simulink model "AMCLIB_FWSpeedLoop_BAM"  (Simulink 9.3)
settings: Solver=VariableStepAuto  StartTime=0.0  StopTime=10.0  RelTol=1e-3
(part 1 of 2)
settings Model: Creator=nxa18952  LastModifiedBy=nxa18952
settings DataIOCC: SaveFormat=Dataset  SignalLoggingSaveFormat=Dataset  ReturnWorkspaceOutputs=on
settings OptimizationCC: LifeSpan=auto
settings DebuggingCC: UnderspecifiedInitializationDetection=Simplified  MergeDetectMultiDrivingBlocksExec=error  FcnCallInpInsideContextMsg=error  SFUnexpectedBacktrackingDiag=error  SFNoUnconditionalDefaultTransitionDiag=error  SFExecutionAtInitializationDiag=warning  ArithmeticOperatorsInVariantConditions=error
settings HardwareCC: ProdBitPerPointer=64  ProdBitPerSizeT=64  ProdBitPerPtrDiffT=64  ProdLargestAtomicFloat=Float  ProdIntDivRoundTo=Zero  ProdEndianess=LittleEndian  ProdWordSize=64  ProdHWDeviceType=Intel->x86-64 (Windows64)
settings ModelReferenceCC: PropagateSignalLabelsOutOfModel=on
settings SFSimCC: SimUseLocalCustomCode=on
settings RTWCC: RTWUseLocalCustomCode=on
settings CodeAppCC: StateflowObjectComments=off
settings GRTTargetCC: TargetLangStandard=C99 (ISO)  CombineOutputUpdateFcns=on  GRTInterface=off
settings ConfigComp: CovMetricSettings=dwe  CovHtmlReporting=off  CovSaveCumulativeToWorkspaceVar=off  CovSaveSingleToWorkspaceVar=off  CovExternalEMLEnable=on

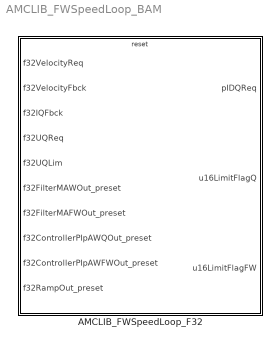
== system AMCLIB_FWSpeedLoop_BAM ==
  AMCLIB_FWSpeedLoop_F32 : Subsystem  TreatAsAtomicUnit=on  mask(AMCLIB_FWSpeedLoop_F32){showStates=Hide (faster execution), resetStatesEnable=Pre-set according to the first set of inputs after reset, showDebugOutputs=Hide, u16NSamplesW=0, u16NSamplesFW=0, f32PropGainQ=0, f32IntegGainQ=0, s16PropGainShiftQ=0, s16IntegGainShiftQ=0, f32LowerLimitQ=0, f32UpperLimitQ=0, f32PropGainFW=0, f32IntegGainFW=0, s16PropGainShiftFW=0, s16IntegGainShiftFW=0, f32LowerLimitFW=0, f32UpperLimitFW=0, f32RampUp=0, f32RampDown=0}
      mask prompts: showStates "Show internal states"; resetStatesEnable "Internal state after reset"; showDebugOutputs "Show debugging outputs"; u16NSamplesW "u16NSamplesW (velocity GDFLIB_FilterMA - recalculated smoothing factor)"; u16NSamplesFW "u16NSamplesFW (FW GDFLIB_FilterMA - recalculated smoothing factor)"; f32PropGainQ "f32PropGainQ (q-axis GFLIB_ControllerPIpAW - proportional gain)"; f32IntegGainQ "f32IntegGainQ (q-axis GFLIB_ControllerPIpAW - integral gain)"; s16PropGainShiftQ "s16PropGainShiftQ (q-axis GFLIB_ControllerPIpAW - scaling bitwise shift applied to the proportional gain)"; s16IntegGainShiftQ "s16IntegGainShiftQ (q-axis GFLIB_ControllerPIpAW - scaling bitwise shift applied to the integral gain)"; f32LowerLimitQ "f32LowerLimitQ (q-axis GFLIB_ControllerPIpAW - lower limit)"; f32UpperLimitQ "f32UpperLimitQ (q-axis GFLIB_ControllerPIpAW - upper limit)"; f32PropGainFW "f32PropGainFW (FW GFLIB_ControllerPIpAW - proportional gain)"; f32IntegGainFW "f32IntegGainFW (FW GFLIB_ControllerPIpAW - integral gain)"; s16PropGainShiftFW "s16PropGainShiftFW (FW GFLIB_ControllerPIpAW - scaling bitwise shift applied to the proportional gain)"; s16IntegGainShiftFW "s16IntegGainShiftFW (FW GFLIB_ControllerPIpAW - scaling bitwise shift applied to the integral gain)"; f32LowerLimitFW "f32LowerLimitFW (FW GFLIB_ControllerPIpAW - lower limit)"; f32UpperLimitFW "f32UpperLimitFW (FW GFLIB_ControllerPIpAW - upper limit)"; f32RampUp "f32RampUp (Ramp up increment coefficient)"; f32RampDown "f32RampDown (Ramp decrement coefficient)"
      mask help: Speed loop controller with Field Weakening capability for the PMSM field-oriented control algorithm in 32-bit fixed-point fractional implementation. This block supports re-initialization of the internal state during simulation. If the block is reset, the outputs of the MA filters, PI controllers, and the ramp will be aligned with the inputs f32FilterMAWOut_preset, f32FilterMAFWOut_preset, f32ControllerPIpAWQOut_preset, f32ControllerPIpAWFWOut_preset, and f32RampOut_preset. Refer to the AMMCLIB User's Guide for further details.
      mask init:
      | if ~evalin('base','exist(''tS8'',''var'')')
      |   if (2 ~= exist('SWLIBS_Typedefs.mat','file'))
      |       error('File SWLIBS_Typedefs.mat is not on the Matlab path. Please add the AMMCLIB "bam" folder in the Matlab Search Path.');
      |   else
      |       evalin('base', 'load(''SWLIBS_Typedefs.mat'')');
      |   end
      | end
      | if showStates == 1
      |     % hidden state variables
      |     if strcmp(get_param([gcb '/u16NSamplesW'], 'BlockType'), 'Inport')
      |         posblk = get_param(gcb, 'Position');
      | 
      |         pos = get_param(    [gcb, '/u16NSamplesW'], 'Position');
      |         orient = get_param( [gcb, '/u16NSamplesW'], 'Orientation');
      |         delete_block(       [gcb, '/u16NSamplesW']);
      |         add_block('built-in/Ground', [gcb, '/u16NSamplesW'], 'Position', pos, 'Orientation', orient);
      | 
      |         pos = get_param(    [gcb, '/u16NSamplesFW'], 'Position');
      |         orient = get_param( [gcb, '/u16NSamplesFW'], 'Orientation');
      |         delete_block(       [gcb, '/u16NSamplesFW']);
      |         add_block('built-in/Ground', [gcb, '/u16NSamplesFW'], 'Position', pos, 'Orientation', orient);
      | 
      |         pos = get_param(    [gcb, '/f32PropGainQ'], 'Position');
      |         orient = get_param( [gcb, '/f32PropGainQ'], 'Orientation');
      |         delete_block(       [gcb, '/f32PropGainQ']);
      |         add_block('built-in/Ground', [gcb, '/f32PropGainQ'], 'Position', pos, 'Orientation', orient);
      | 
      |         pos = get_param(    [gcb, '/f32IntegGainQ'], 'Position');
      |         orient = get_param( [gcb, '/f32IntegGainQ'], 'Orientation');
      |         delete_block(       [gcb, '/f32IntegGainQ']);
      |         add_block('built-in/Ground', [gcb, '/f32IntegGainQ'], 'Position', pos, 'Orientation', orient);
      | 
      |         pos = get_param(    [gcb, '/s16PropGainShiftQ'], 'Position');
      |         orient = get_param( [gcb, '/s16PropGainShiftQ'], 'Orientation');
      |         delete_block(       [gcb, '/s16PropGainShiftQ']);
      |         add_block('built-in/Ground', [gcb, '/s16PropGainShiftQ'], 'Position', pos, 'Orientation', orient);
      | 
      |         pos = get_param(    [gcb, '/s16IntegGainShiftQ'], 'Position');
      |         orient = get_param( [gcb, '/s16IntegGainShiftQ'], 'Orientation');
      |         delete_block(       [gcb, '/s16IntegGainShiftQ']);
      |         add_block('built-in/Ground', [gcb, '/s16IntegGainShiftQ'], 'Position', pos, 'Orientation', orient);
      | 
      |         pos = get_param(    [gcb, '/f32LowerLimitQ'], 'Position');
      |         orient = get_param( [gcb, '/f32LowerLimitQ'], 'Orientation');
      |         delete_block(       [gcb, '/f32LowerLimitQ']);
      |         add_block('built-in/Ground', [gcb, '/f32LowerLimitQ'], 'Position', pos, 'Orientation', orient);
      | 
      |         pos = get_param(    [gcb, '/f32UpperLimitQ'], 'Position');
      |         orient = get_param( [gcb, '/f32UpperLimitQ'], 'Orientation');
      |         delete_block(       [gcb, '/f32UpperLimitQ']);
      |         add_block('built-in/Ground', [gcb, '/f32UpperLimitQ'], 'Position', pos, 'Orientation', orient);
      | 
      |         pos = get_param(    [gcb, '/f32PropGainFW'], 'Position');
      |         orient = get_param( [gcb, '/f32PropGainFW'], 'Orientation');
      |         delete_block(       [gcb, '/f32PropGainFW']);
      |         add_block('built-in/Ground', [gcb, '/f32PropGainFW'], 'Position', pos, 'Orientation', orient);
      | 
      |         pos = get_param(    [gcb, '/f32IntegGainFW'], 'Position');
      |         orient = get_param( [gcb, '/f32IntegGainFW'], 'Orientation');
      |         delete_block(       [gcb, '/f32IntegGainFW']);
      |         add_block('built-in/Ground', [gcb, '/f32IntegGainFW'], 'Position', pos, 'Orientation', orient);
      | 
      |         pos = get_param(    [gcb, '/s16PropGainShiftFW'], 'Position');
      |         orient = get_param( [gcb, '/s16PropGainShiftFW'], 'Orientation');
      |         delete_block(       [gcb, '/s16PropGainShiftFW']);
      |         add_block('built-in/Ground', [gcb, '/s16PropGainShiftFW'], 'Position', pos, 'Orientation', orient);
      | 
      |         pos = get_param(    [gcb, '/s16IntegGainShiftFW'], 'Position');
      |         orient = get_param( [gcb, '/s16IntegGainShiftFW'], 'Orientation');
      |         delete_block(       [gcb, '/s16IntegGainShiftFW']);
      |         add_block('built-in/Ground', [gcb, '/s16IntegGainShiftFW'], 'Position', pos, 'Orientation', orient);
      | 
      |         pos = get_param(    [gcb, '/f32LowerLimitFW'], 'Position');
      |         orient = get_param( [gcb, '/f32LowerLimitFW'], 'Orientation');
      |         delete_block(       [gcb, '/f32LowerLimitFW']);
      |         add_block('built-in/Ground', [gcb, '/f32LowerLimitFW'], 'Position', pos, 'Orientation', orient);
      | 
      |         pos = get_param(    [gcb, '/f32UpperLimitFW'], 'Position');
      |         orient = get_param( [gcb, '/f32UpperLimitFW'], 'Orientation');
      |         delete_block(       [gcb, '/f32UpperLimitFW']);
      |         add_block('built-in/Ground', [gcb, '/f32UpperLimitFW'], 'Position', pos, 'Orientation', orient);
      | 
      |         pos = get_param(    [gcb, '/f32RampUp'], 'Position');
      |         orient = get_param( [gcb, '/f32RampUp'], 'Orientation');
      |         delete_block(       [gcb, '/f32RampUp']);
      |         add_block('built-in/Ground', [gcb, '/f32RampUp'], 'Position', pos, 'Orientation', orient);
      | 
      |         pos = get_param(    [gcb, '/f32RampDown'], 'Position');
      |         orient = get_param( [gcb, '/f32RampDown'], 'Orientation');
      |         delete_block(       [gcb, '/f32RampDown']);
      |         add_block('built-in/Ground', [gcb, '/f32RampDown'], 'Position', pos, 'Orientation', orient);
      | 
      |         pos = get_param(    [gcb, '/f32IQReqK_1'], 'Position');
      |         orient = get_param( [gcb, '/f32IQReqK_1'], 'Orientation');
      |         delete_block(       [gcb, '/f32IQReqK_1']);
      |         add_block('built-in/Ground', [gcb, '/f32IQReqK_1'], 'Position', pos, 'Orientation', orient);
      | 
      |         pos = get_param(    [gcb, '/f32AccW'], 'Position');
      |         orient = get_param( [gcb, '/f32AccW'], 'Orientation');
      |         delete_block(       [gcb, '/f32AccW']);
      |         add_block('built-in/Ground', [gcb, '/f32AccW'], 'Position', pos, 'Orientation', orient);
      | 
      |         pos = get_param(    [gcb, '/f32AccFW'], 'Position');
      |         orient = get_param( [gcb, '/f32AccFW'], 'Orientation');
      |         delete_block(       [gcb, '/f32AccFW']);
      |         add_block('built-in/Ground', [gcb, '/f32AccFW'], 'Position', pos, 'Orientation', orient);
      | 
      |         pos = get_param(    [gcb, '/f32IntegPartK_1Q'], 'Position');
      |         orient = get_param( [gcb, '/f32IntegPartK_1Q'], 'Orientation');
      |         delete_block(       [gcb, '/f32IntegPartK_1Q']);
      |         add_block('built-in/Ground', [gcb, '/f32IntegPartK_1Q'], 'Position', pos, 'Orientation', orient);
      | 
      |         pos = get_param(    [gcb, '/f32InK_1Q'], 'Position');
      |         orient = get_param( [gcb, '/f32InK_1Q'], 'Orientation');
      |         delete_block(       [gcb, '/f32InK_1Q']);
      |         add_block('built-in/Ground', [gcb, '/f32InK_1Q'], 'Position', pos, 'Orientation', orient);
      | 
      |         pos = get_param(    [gcb, '/f32IntegPartK_1FW'], 'Position');
      |         orient = get_param( [gcb, '/f32IntegPartK_1FW'], 'Orientation');
      |         delete_block(       [gcb, '/f32IntegPartK_1FW']);
      |         add_block('built-in/Ground', [gcb, '/f32IntegPartK_1FW'], 'Position', pos, 'Orientation', orient);
      | 
      |         pos = get_param(    [gcb, '/f32InK_1FW'], 'Position');
      |         orient = get_param( [gcb, '/f32InK_1FW'], 'Orientation');
      |         delete_block(       [gcb, '/f32InK_1FW']);
      |         add_block('built-in/Ground', [gcb, '/f32InK_1FW'], 'Position', pos, 'Orientation', orient);
      | 
      |         pos = get_param(    [gcb, '/f32State'], 'Position');
      |         orient = get_param( [gcb, '/f32State'], 'Orientation');
      |         delete_block(       [gcb, '/f32State']);
      |         add_block('built-in/Ground', [gcb, '/f32State'], 'Position', pos, 'Orientation', orient);
      | 
      | 
      |         pos = get_param(    [gcb '/f32AccW_Out'], 'Position');
      |         orient = get_param( [gcb '/f32AccW_Out'], 'Orientation');
      |         delete_block(       [gcb '/f32AccW_Out']);
      |         add_block('built-in/Terminator', [gcb '/f32AccW_Out'], 'Position', pos, 'Orientation', orient);
      | 
      |         pos = get_param(    [gcb '/f32AccFW_Out'], 'Position');
      |         orient = get_param( [gcb '/f32AccFW_Out'], 'Orientation');
      |         delete_block(       [gcb '/f32AccFW_Out']);
      |         add_block('built-in/Terminator', [gcb '/f32AccFW_Out'], 'Position', pos, 'Orientation', orient);
      | 
      |         pos = get_param(    [gcb '/f32IntegPartK_1Q_Out'], 'Position');
      |         orient = get_param( [gcb '/f32IntegPartK_1Q_Out'], 'Orientation');
      |         delete_block(       [gcb '/f32IntegPartK_1Q_Out']);
      |         add_block('built-in/Terminator', [gcb '/f32IntegPartK_1Q_Out'], 'Position', pos, 'Orientation', orient);
      | 
      |         pos = get_param(    [gcb '/f32InK_1Q_Out'], 'Position');
      |         orient = get_param( [gcb '/f32InK_1Q_Out'], 'Orientation');
      |         delete_block(       [gcb '/f32InK_1Q_Out']);
      |         add_block('built-in/Terminator', [gcb '/f32InK_1Q_Out'], 'Position', pos, 'Orientation', orient);
      | 
      |         pos = get_param(    [gcb '/f32IntegPartK_1FW_Out'], 'Position');
      |         orient = get_param( [gcb '/f32IntegPartK_1FW_Out'], 'Orientation');
      |         delete_block(       [gcb '/f32IntegPartK_1FW_Out']);
      |         add_block('built-in/Terminator', [gcb '/f32IntegPartK_1FW_Out'], 'Position', pos, 'Orientation', orient);
      | 
      |         pos = get_param(    [gcb '/f32InK_1FW_Out'], 'Position');
      |         orient = get_param( [gcb '/f32InK_1FW_Out'], 'Orientation');
      |         delete_block(       [gcb '/f32InK_1FW_Out']);
      |         add_block('built-in/Terminator', [gcb '/f32InK_1FW_Out'], 'Position', pos, 'Orientation', orient);
      | 
      |         pos = get_param(    [gcb '/f32State_Out'], 'Position');
      |         orient = get_param( [gcb '/f32State_Out'], 'Orientation');
      |         delete_block(       [gcb '/f32State_Out']);
      |         add_block('built-in/Terminator', [gcb '/f32State_Out'], 'Position', pos, 'Orientation', orient);
      | 
      | 
      |         if strcmp(get_param([gcb '/f32WReqFilt'], 'BlockType'), 'Outport')
      |             pos = get_param(    [gcb '/f32WReqFilt'], 'Position');
      |             orient = get_param( [gcb '/f32WReqFilt'], 'Orientation');
      |             delete_block(       [gcb '/f32WReqFilt']);
      |             add_block('built-in/Terminator', [gcb '/f32WReqFilt'], 'Position', pos, 'Orientation', orient);
      | 
      |             pos = get_param(    [gcb '/f32WErr'], 'Position');
      |             orient = get_param( [gcb '/f32WErr'], 'Orientation');
      |             delete_block(       [gcb '/f32WErr']);
      |             add_block('built-in/Terminator', [gcb '/f32WErr'], 'Position', pos, 'Orientation', orient);
      | 
      |             pos = get_param(    [gcb '/f32WFbckFilt'], 'Position');
      |             orient = get_param( [gcb '/f32WFbckFilt'], 'Orientation');
      |             delete_block(       [gcb '/f32WFbckFilt']);
      |             add_block('built-in/Terminator', [gcb '/f32WFbckFilt'], 'Position', pos, 'Orientation', orient);
      | 
      |             pos = get_param(    [gcb '/f32IDQReqAmp'], 'Position');
      |             orient = get_param( [gcb '/f32IDQReqAmp'], 'Orientation');
      |             delete_block(       [gcb '/f32IDQReqAmp']);
      |             add_block('built-in/Terminator', [gcb '/f32IDQReqAmp'], 'Position', pos, 'Orientation', orient);
      | 
      |             pos = get_param(    [gcb '/f32IQErrSign'], 'Position');
      |             orient = get_param( [gcb '/f32IQErrSign'], 'Orientation');
      |             delete_block(       [gcb '/f32IQErrSign']);
      |             add_block('built-in/Terminator', [gcb '/f32IQErrSign'], 'Position', pos, 'Orientation', orient);
      | 
      |             pos = get_param(    [gcb '/f32IQErr'], 'Position');
      |             orient = get_param( [gcb '/f32IQErr'], 'Orientation');
      |             delete_block(       [gcb '/f32IQErr']);
      |             add_block('built-in/Terminator', [gcb '/f32IQErr'], 'Position', pos, 'Orientation', orient);
      | 
      |             pos = get_param(    [gcb '/f32FWErr'], 'Position');
      |             orient = get_param( [gcb '/f32FWErr'], 'Orientation');
      |             delete_block(       [gcb '/f32FWErr']);
      |             add_block('built-in/Terminator', [gcb '/f32FWErr'], 'Position', pos, 'Orientation', orient);
      | 
      |             pos = get_param(    [gcb '/f32UQErr'], 'Position');
      |             orient = get_param( [gcb '/f32UQErr'], 'Orientation');
      |             delete_block(       [gcb '/f32UQErr']);
      |             add_block('built-in/Terminator', [gcb '/f32UQErr'], 'Position', pos, 'Orientation', orient);
      | 
      |             pos = get_param(    [gcb '/f32FWErrFilt'], 'Position');
      |             orient = get_param( [gcb '/f32FWErrFilt'], 'Orientation');
      |             delete_block(       [gcb '/f32FWErrFilt']);
      |             add_block('built-in/Terminator', [gcb '/f32FWErrFilt'], 'Position', pos, 'Orientation', orient);
      | 
      |             pos = get_param(    [gcb '/f32FWAngle'], 'Position');
      |             orient = get_param( [gcb '/f32FWAngle'], 'Orientation');
      |             delete_block(       [gcb '/f32FWAngle']);
      |             add_block('built-in/Terminator', [gcb '/f32FWAngle'], 'Position', pos, 'Orientation', orient);
      | 
      |             pos = get_param(    [gcb '/f32FWSin'], 'Position');
      |             orient = get_param( [gcb '/f32FWSin'], 'Orientation');
      |             delete_block(       [gcb '/f32FWSin']);
      |             add_block('built-in/Terminator', [gcb '/f32FWSin'], 'Position', pos, 'Orientation', orient);
      | 
      |             pos = get_param(    [gcb '/f32FWCos'], 'Position');
      |             orient = get_param( [gcb '/f32FWCos'], 'Orientation');
      |             delete_block(       [gcb '/f32FWCos']);
      |             add_block('built-in/Terminator', [gcb '/f32FWCos'], 'Position', pos, 'Orientation', orient);
      | 
      |         end
      | 
      |         set_param([gcb '/f32VelocityReq'], 'Port', '1');
      |         set_param([gcb '/f32VelocityFbck'], 'Port', '2');
      |         set_param([gcb '/f32IQFbck'], 'Port', '3');
      |         set_param([gcb '/f32UQReq'], 'Port', '4');
      |         set_param([gcb '/f32UQLim'], 'Port', '5');
      |         set_param([gcb '/f32FilterMAWOut_preset'], 'Port', '6');
      |         set_param([gcb '/f32FilterMAFWOut_preset'], 'Port', '7');
      |         set_param([gcb '/f32ControllerPIpAWQOut_preset'], 'Port', '8');
      |         set_param([gcb '/f32ControllerPIpAWFWOut_preset'], 'Port', '9');
      |         set_param([gcb '/f32RampOut_preset'], 'Port', '10');
      | 
      |         set_param([gcb '/pIDQReq'], 'Port', '1');
      |         set_param([gcb '/u16LimitFlagQ'], 'Port', '2');
      |         set_param([gcb '/u16LimitFlagFW'], 'Port', '3');
      | 
      |         set_param(gcb,'MaskEnables',{'on','on','off','on','on','on','on','on','on','on','on','on','on','on','on','on','on','on','on'});
      | 
      |         if (posblk(4) - posblk(2)) > 275
      |           height = 275;
      |           set_param(gcb,'Position',[posblk(1), posblk(2), posblk(3), posblk(2)+height])
      |         end
      |     end
      | else
      |     % shown state variables
      |     if strcmp(get_param([gcb '/u16NSamplesW'], 'BlockType'), 'Ground')
      |         posblk = get_param(gcb, 'Position');
      | 
      |         pos = get_param(    [gcb, '/u16NSamplesW'], 'Position');
      |         orient = get_param( [gcb, '/u16NSamplesW'], 'Orientation');
      |         delete_block(       [gcb, '/u16NSamplesW']);
      |         add_block('built-in/Inport', [gcb, '/u16NSamplesW'], 'Position', pos, 'Orientation', orient, 'OutDataTypeStr', 'uint16');
      | 
      |         pos = get_param(    [gcb, '/u16NSamplesFW'], 'Position');
      |         orient = get_param( [gcb, '/u16NSamplesFW'], 'Orientation');
      |         delete_block(       [gcb, '/u16NSamplesFW']);
      |         add_block('built-in/Inport', [gcb, '/u16NSamplesFW'], 'Position', pos, 'Orientation', orient, 'OutDataTypeStr', 'uint16');
      | 
      |         pos = get_param(    [gcb, '/f32PropGainQ'], 'Position');
      |         orient = get_param( [gcb, '/f32PropGainQ'], 'Orientation');
      |         delete_block(       [gcb, '/f32PropGainQ']);
      |         add_block('built-in/Inport', [gcb, '/f32PropGainQ'], 'Position', pos, 'Orientation', orient, 'OutDataTypeStr', 'int32');
      | 
      |         pos = get_param(    [gcb, '/f32IntegGainQ'], 'Position');
      |         orient = get_param( [gcb, '/f32IntegGainQ'], 'Orientation');
      |         delete_block(       [gcb, '/f32IntegGainQ']);
      |         add_block('built-in/Inport', [gcb, '/f32IntegGainQ'], 'Position', pos, 'Orientation', orient, 'OutDataTypeStr', 'int32');
      | 
      |         pos = get_param(    [gcb, '/s16PropGainShiftQ'], 'Position');
      |         orient = get_param( [gcb, '/s16PropGainShiftQ'], 'Orientation');
      |         delete_block(       [gcb, '/s16PropGainShiftQ']);
      |         add_block('built-in/Inport', [gcb, '/s16PropGainShiftQ'], 'Position', pos, 'Orientation', orient, 'OutDataTypeStr', 'int16');
      | 
      |         pos = get_param(    [gcb, '/s16IntegGainShiftQ'], 'Position');
      |         orient = get_param( [gcb, '/s16IntegGainShiftQ'], 'Orientation');
      |         delete_block(       [gcb, '/s16IntegGainShiftQ']);
      |         add_block('built-in/Inport', [gcb, '/s16IntegGainShiftQ'], 'Position', pos, 'Orientation', orient, 'OutDataTypeStr', 'int16');
      | 
      |         pos = get_param(    [gcb, '/f32LowerLimitQ'], 'Position');
      |         orient = get_param( [gcb, '/f32LowerLimitQ'], 'Orientation');
      |         delete_block(       [gcb, '/f32LowerLimitQ']);
      |         add_block('built-in/Inport', [gcb, '/f32LowerLimitQ'], 'Position', pos, 'Orientation', orient, 'OutDataTypeStr', 'int32');
      | 
      |         pos = get_param(    [gcb, '/f32UpperLimitQ'], 'Position');
      |         orient = get_param( [gcb, '/f32UpperLimitQ'], 'Orientation');
      |         delete_block(       [gcb, '/f32UpperLimitQ']);
      |         add_block('built-in/Inport', [gcb, '/f32UpperLimitQ'], 'Position', pos, 'Orientation', orient, 'OutDataTypeStr', 'int32');
      | 
      |         pos = get_param(    [gcb, '/f32PropGainFW'], 'Position');
      |         orient = get_param( [gcb, '/f32PropGainFW'], 'Orientation');
      |         delete_block(       [gcb, '/f32PropGainFW']);
      |         add_block('built-in/Inport', [gcb, '/f32PropGainFW'], 'Position', pos, 'Orientation', orient, 'OutDataTypeStr', 'int32');
      | 
      |         pos = get_param(    [gcb, '/f32IntegGainFW'], 'Position');
      |         orient = get_param( [gcb, '/f32IntegGainFW'], 'Orientation');
      |         delete_block(       [gcb, '/f32IntegGainFW']);
      |         add_block('built-in/Inport', [gcb, '/f32IntegGainFW'], 'Position', pos, 'Orientation', orient, 'OutDataTypeStr', 'int32');
      | 
      |         pos = get_param(    [gcb, '/s16PropGainShiftFW'], 'Position');
      |         orient = get_param( [gcb, '/s16PropGainShiftFW'], 'Orientation');
      |         delete_block(       [gcb, '/s16PropGainShiftFW']);
      |         add_block('built-in/Inport', [gcb, '/s16PropGainShiftFW'], 'Position', pos, 'Orientation', orient, 'OutDataTypeStr', 'int16');
      | 
      |         pos = get_param(    [gcb, '/s16IntegGainShiftFW'], 'Position');
      |         orient = get_param( [gcb, '/s16IntegGainShiftFW'], 'Orientation');
      |         delete_block(       [gcb, '/s16IntegGainShiftFW']);
      |         add_block('built-in/Inport', [gcb, '/s16IntegGainShiftFW'], 'Position', pos, 'Orientation', orient, 'OutDataTypeStr', 'int16');
      | 
      |         pos = get_param(    [gcb, '/f32LowerLimitFW'], 'Position');
      |         orient = get_param( [gcb, '/f32LowerLimitFW'], 'Orientation');
      |         delete_block(       [gcb, '/f32LowerLimitFW']);
      |         add_block('built-in/Inport', [gcb, '/f32LowerLimitFW'], 'Position', pos, 'Orientation', orient, 'OutDataTypeStr', 'int32');
      | 
      |         pos = get_param(    [gcb, '/f32UpperLimitFW'], 'Position');
      |         orient = get_param( [gcb, '/f32UpperLimitFW'], 'Orientation');
      |         delete_block(       [gcb, '/f32UpperLimitFW']);
      |         add_block('built-in/Inport', [gcb, '/f32UpperLimitFW'], 'Position', pos, 'Orientation', orient, 'OutDataTypeStr', 'int32');
      | 
      |         pos = get_param(    [gcb, '/f32RampUp'], 'Position');
      |         orient = get_param( [gcb, '/f32RampUp'], 'Orientation');
      |         delete_block(       [gcb, '/f32RampUp']);
      |         add_block('built-in/Inport', [gcb, '/f32RampUp'], 'Position', pos, 'Orientation', orient, 'OutDataTypeStr', 'int32');
      | 
      |         pos = get_param(    [gcb, '/f32RampDown'], 'Position');
      |         orient = get_param( [gcb, '/f32RampDown'], 'Orientation');
      |         delete_block(       [gcb, '/f32RampDown']);
      |         add_block('built-in/Inport', [gcb, '/f32RampDown'], 'Position', pos, 'Orientation', orient, 'OutDataTypeStr', 'int32');
      | 
      |         pos = get_param(    [gcb, '/f32IQReqK_1'], 'Position');
      |         orient = get_param( [gcb, '/f32IQReqK_1'], 'Orientation');
      |         delete_block(       [gcb, '/f32IQReqK_1']);
      |         add_block('built-in/Inport', [gcb, '/f32IQReqK_1'], 'Position', pos, 'Orientation', orient, 'OutDataTypeStr', 'int32');
      | 
      |         pos = get_param(    [gcb, '/f32AccW'], 'Position');
      |         orient = get_param( [gcb, '/f32AccW'], 'Orientation');
      |         delete_block(       [gcb, '/f32AccW']);
      |         add_block('built-in/Inport', [gcb, '/f32AccW'], 'Position', pos, 'Orientation', orient, 'OutDataTypeStr', 'int32');
      | 
      |         pos = get_param(    [gcb, '/f32AccFW'], 'Position');
      |         orient = get_param( [gcb, '/f32AccFW'], 'Orientation');
      |         delete_block(       [gcb, '/f32AccFW']);
      |         add_block('built-in/Inport', [gcb, '/f32AccFW'], 'Position', pos, 'Orientation', orient, 'OutDataTypeStr', 'int32');
      | 
      |         pos = get_param(    [gcb, '/f32IntegPartK_1Q'], 'Position');
      |         orient = get_param( [gcb, '/f32IntegPartK_1Q'], 'Orientation');
      |         delete_block(       [gcb, '/f32IntegPartK_1Q']);
      |         add_block('built-in/Inport', [gcb, '/f32IntegPartK_1Q'], 'Position', pos, 'Orientation', orient, 'OutDataTypeStr', 'int32');
      | 
      |         pos = get_param(    [gcb, '/f32InK_1Q'], 'Position');
      |         orient = get_param( [gcb, '/f32InK_1Q'], 'Orientation');
      |         delete_block(       [gcb, '/f32InK_1Q']);
      |         add_block('built-in/Inport', [gcb, '/f32InK_1Q'], 'Position', pos, 'Orientation', orient, 'OutDataTypeStr', 'int32');
      | 
      |         pos = get_param(    [gcb, '/f32IntegPartK_1FW'], 'Position');
      |         orient = get_param( [gcb, '/f32IntegPartK_1FW'], 'Orientation');
      |         delete_block(       [gcb, '/f32IntegPartK_1FW']);
      |         add_block('built-in/Inport', [gcb, '/f32IntegPartK_1FW'], 'Position', pos, 'Orientation', orient, 'OutDataTypeStr', 'int32');
      | 
      |         pos = get_param(    [gcb, '/f32InK_1FW'], 'Position');
      |         orient = get_param( [gcb, '/f32InK_1FW'], 'Orientation');
      |         delete_block(       [gcb, '/f32InK_1FW']);
      |         add_block('built-in/Inport', [gcb, '/f32InK_1FW'], 'Position', pos, 'Orientation', orient, 'OutDataTypeStr', 'int32');
      | 
      |         pos = get_param(    [gcb, '/f32State'], 'Position');
      |         orient = get_param( [gcb, '/f32State'], 'Orientation');
      |         delete_block(       [gcb, '/f32State']);
      |         add_block('built-in/Inport', [gcb, '/f32State'], 'Position', pos, 'Orientation', orient, 'OutDataTypeStr', 'int32');
      | 
      | 
      |         pos = get_param(    [gcb '/f32AccW_Out'], 'Position');
      |         orient = get_param( [gcb '/f32AccW_Out'], 'Orientation');
      |         delete_block(       [gcb '/f32AccW_Out']);
      |         add_block('built-in/Outport', [gcb '/f32AccW_Out'], 'Position', pos, 'Orientation', orient);
      | 
      |         pos = get_param(    [gcb '/f32AccFW_Out'], 'Position');
      |         orient = get_param( [gcb '/f32AccFW_Out'], 'Orientation');
      |         delete_block(       [gcb '/f32AccFW_Out']);
      |         add_block('built-in/Outport', [gcb '/f32AccFW_Out'], 'Position', pos, 'Orientation', orient);
      | 
      |         pos = get_param(    [gcb '/f32IntegPartK_1Q_Out'], 'Position');
      |         orient = get_param( [gcb '/f32IntegPartK_1Q_Out'], 'Orientation');
      |         delete_block(       [gcb '/f32IntegPartK_1Q_Out']);
      |         add_block('built-in/Outport', [gcb '/f32IntegPartK_1Q_Out'], 'Position', pos, 'Orientation', orient);
      | 
      |         pos = get_param(    [gcb '/f32InK_1Q_Out'], 'Position');
      |         orient = get_param( [gcb '/f32InK_1Q_Out'], 'Orientation');
      |         delete_block(       [gcb '/f32InK_1Q_Out']);
      |         add_block('built-in/Outport', [gcb '/f32InK_1Q_Out'], 'Position', pos, 'Orientation', orient);
      | 
      |         pos = get_param(    [gcb '/f32IntegPartK_1FW_Out'], 'Position');
      |         orient = get_param( [gcb '/f32IntegPartK_1FW_Out'], 'Orientation');
      |         delete_block(       [gcb '/f32IntegPartK_1FW_Out']);
      |         add_block('built-in/Outport', [gcb '/f32IntegPartK_1FW_Out'], 'Position', pos, 'Orientation', orient);
      | 
      |         pos = get_param(    [gcb '/f32InK_1FW_Out'], 'Position');
      |         orient = get_param( [gcb '/f32InK_1FW_Out'], 'Orientation');
      |         delete_block(       [gcb '/f32InK_1FW_Out']);
      |         add_block('built-in/Outport', [gcb '/f32InK_1FW_Out'], 'Position', pos, 'Orientation', orient);
      | 
      |         pos = get_param(    [gcb '/f32State_Out'], 'Position');
      |         orient = get_param( [gcb '/f32State_Out'], 'Orientation');
      |         delete_block(       [gcb '/f32State_Out']);
      |         add_block('built-in/Outport', [gcb '/f32State_Out'], 'Position', pos, 'Orientation', orient);
      | 
      | 
      |         if (showDebugOutputs == 2) && (strcmp(get_param([gcb '/f32WReqFilt'], 'BlockType'), 'Terminator'))
      |             pos = get_param(    [gcb '/f32WReqFilt'], 'Position');
      |             orient = get_param( [gcb '/f32WReqFilt'], 'Orientation');
      |             delete_block(       [gcb '/f32WReqFilt']);
      |             add_block('built-in/Outport', [gcb '/f32WReqFilt'], 'Position', pos, 'Orientation', orient);
      | 
      |             pos = get_param(    [gcb '/f32WErr'], 'Position');
      |             orient = get_param( [gcb '/f32WErr'], 'Orientation');
      |             delete_block(       [gcb '/f32WErr']);
      |             add_block('built-in/Outport', [gcb '/f32WErr'], 'Position', pos, 'Orientation', orient);
      | 
      |             pos = get_param(    [gcb '/f32WFbckFilt'], 'Position');
      |             orient = get_param( [gcb '/f32WFbckFilt'], 'Orientation');
      |             delete_block(       [gcb '/f32WFbckFilt']);
      |             add_block('built-in/Outport', [gcb '/f32WFbckFilt'], 'Position', pos, 'Orientation', orient);
      | 
      |             pos = get_param(    [gcb '/f32IDQReqAmp'], 'Position');
      |             orient = get_param( [gcb '/f32IDQReqAmp'], 'Orientation');
      |             delete_block(       [gcb '/f32IDQReqAmp']);
      |             add_block('built-in/Outport', [gcb '/f32IDQReqAmp'], 'Position', pos, 'Orientation', orient);
      | 
      |             pos = get_param(    [gcb '/f32IQErrSign'], 'Position');
      |             orient = get_param( [gcb '/f32IQErrSign'], 'Orientation');
      |             delete_block(       [gcb '/f32IQErrSign']);
      |             add_block('built-in/Outport', [gcb '/f32IQErrSign'], 'Position', pos, 'Orientation', orient);
      | 
      |             pos = get_param(    [gcb '/f32IQErr'], 'Position');
      |             orient = get_param( [gcb '/f32IQErr'], 'Orientation');
      |             delete_block(       [gcb '/f32IQErr']);
      |             add_block('built-in/Outport', [gcb '/f32IQErr'], 'Position', pos, 'Orientation', orient);
      | 
      |             pos = get_param(    [gcb '/f32FWErr'], 'Position');
      |             orient = get_param( [gcb '/f32FWErr'], 'Orientation');
      |             delete_block(       [gcb '/f32FWErr']);
      |             add_block('built-in/Outport', [gcb '/f32FWErr'], 'Position', pos, 'Orientation', orient);
      | 
      |             pos = get_param(    [gcb '/f32UQErr'], 'Position');
      |             orient = get_param( [gcb '/f32UQErr'], 'Orientation');
      |             delete_block(       [gcb '/f32UQErr']);
      |             add_block('built-in/Outport', [gcb '/f32UQErr'], 'Position', pos, 'Orientation', orient);
      | 
      |             pos = get_param(    [gcb '/f32FWErrFilt'], 'Position');
      |             orient = get_param( [gcb '/f32FWErrFilt'], 'Orientation');
      |             delete_block(       [gcb '/f32FWErrFilt']);
      |             add_block('built-in/Outport', [gcb '/f32FWErrFilt'], 'Position', pos, 'Orientation', orient);
      | 
      |             pos = get_param(    [gcb '/f32FWAngle'], 'Position');
      |             orient = get_param( [gcb '/f32FWAngle'], 'Orientation');
      |             delete_block(       [gcb '/f32FWAngle']);
      |             add_block('built-in/Outport', [gcb '/f32FWAngle'], 'Position', pos, 'Orientation', orient);
      | 
      |             pos = get_param(    [gcb '/f32FWSin'], 'Position');
      |             orient = get_param( [gcb '/f32FWSin'], 'Orientation');
      |             delete_block(       [gcb '/f32FWSin']);
      |             add_block('built-in/Outport', [gcb '/f32FWSin'], 'Position', pos, 'Orientation', orient);
      | 
      |             pos = get_param(    [gcb '/f32FWCos'], 'Position');
      |             orient = get_param( [gcb '/f32FWCos'], 'Orientation');
      |             delete_block(       [gcb '/f32FWCos']);
      |             add_block('built-in/Outport', [gcb '/f32FWCos'], 'Position', pos, 'Orientation', orient);
      | 
      |         end
      | 
      |         set_param([gcb '/f32VelocityReq'], 'Port', '1');
      |         set_param([gcb '/f32VelocityFbck'], 'Port', '2');
      |         set_param([gcb '/f32IQFbck'], 'Port', '3');
      |         set_param([gcb '/f32UQReq'], 'Port', '4');
      |         set_param([gcb '/f32UQLim'], 'Port', '5');
      |         set_param([gcb '/f32FilterMAWOut_preset'], 'Port', '6');
      |         set_param([gcb '/f32FilterMAFWOut_preset'], 'Port', '7');
      |         set_param([gcb '/f32ControllerPIpAWQOut_preset'], 'Port', '8');
      |         set_param([gcb '/f32ControllerPIpAWFWOut_preset'], 'Port', '9');
      |         set_param([gcb '/f32RampOut_preset'], 'Port', '10');
      |         set_param([gcb '/u16NSamplesW'], 'Port', '11');
      |         set_param([gcb '/u16NSamplesFW'], 'Port', '12');
      |         set_param([gcb '/f32PropGainQ'], 'Port', '13');
      |         set_param([gcb '/f32IntegGainQ'], 'Port', '14');
      |         set_param([gcb '/s16PropGainShiftQ'], 'Port', '15');
      |         set_param([gcb '/s16IntegGainShiftQ'], 'Port', '16');
      |         set_param([gcb '/f32LowerLimitQ'], 'Port', '17');
      |         set_param([gcb '/f32UpperLimitQ'], 'Port', '18');
      |         set_param([gcb '/f32PropGainFW'], 'Port', '19');
      |         set_param([gcb '/f32IntegGainFW'], 'Port', '20');
      |         set_param([gcb '/s16PropGainShiftFW'], 'Port', '21');
      |         set_param([gcb '/s16IntegGainShiftFW'], 'Port', '22');
      |         set_param([gcb '/f32LowerLimitFW'], 'Port', '23');
      |         set_param([gcb '/f32UpperLimitFW'], 'Port', '24');
      |         set_param([gcb '/f32RampUp'], 'Port', '25');
      |         set_param([gcb '/f32RampDown'], 'Port', '26');
      |         set_param([gcb '/f32IQReqK_1'], 'Port', '27');
      |         set_param([gcb '/f32AccW'], 'Port', '28');
      |         set_param([gcb '/f32AccFW'], 'Port', '29');
      |         set_param([gcb '/f32IntegPartK_1Q'], 'Port', '30');
      |         set_param([gcb '/f32InK_1Q'], 'Port', '31');
      |         set_param([gcb '/f32IntegPartK_1FW'], 'Port', '32');
      |         set_param([gcb '/f32InK_1FW'], 'Port', '33');
      |         set_param([gcb '/f32State'], 'Port', '34');
      | 
      |         if (showDebugOutputs == 2)
      |             set_param([gcb '/pIDQReq'], 'Port', '1');
      |             set_param([gcb '/u16LimitFlagQ'], 'Port', '2');
      |             set_param([gcb '/u16LimitFlagFW'], 'Port', '3');
      |             set_param([gcb '/f32WReqFilt'], 'Port', '4');
      |             set_param([gcb '/f32WErr'], 'Port', '5');
      |             set_param([gcb '/f32WFbckFilt'], 'Port', '6');
      |             set_param([gcb '/f32IDQReqAmp'], 'Port', '7');
      |             set_param([gcb '/f32IQErrSign'], 'Port', '8');
      |             set_param([gcb '/f32IQErr'], 'Port', '9');
      |             set_param([gcb '/f32FWErr'], 'Port', '10');
      |             set_param([gcb '/f32UQErr'], 'Port', '11');
      |             set_param([gcb '/f32FWErrFilt'], 'Port', '12');
      |             set_param([gcb '/f32FWAngle'], 'Port', '13');
      |             set_param([gcb '/f32FWSin'], 'Port', '14');
      |             set_param([gcb '/f32FWCos'], 'Port', '15');
      |             set_param([gcb '/f32AccW_Out'], 'Port', '16');
      |             set_param([gcb '/f32AccFW_Out'], 'Port', '17');
      |             set_param([gcb '/f32IntegPartK_1Q_Out'], 'Port', '18');
      |             set_param([gcb '/f32InK_1Q_Out'], 'Port', '19');
      |             set_param([gcb '/f32IntegPartK_1FW_Out'], 'Port', '20');
      |             set_param([gcb '/f32InK_1FW_Out'], 'Port', '21');
      |             set_param([gcb '/f32State_Out'], 'Port', '22');
      |         else
      |             set_param([gcb '/pIDQReq'], 'Port', '1');
      |             set_param([gcb '/u16LimitFlagQ'], 'Port', '2');
      |             set_param([gcb '/u16LimitFlagFW'], 'Port', '3');
      |             set_param([gcb '/f32AccW_Out'], 'Port', '4');
      |             set_param([gcb '/f32AccFW_Out'], 'Port', '5');
      |             set_param([gcb '/f32IntegPartK_1Q_Out'], 'Port', '6');
      |             set_param([gcb '/f32InK_1Q_Out'], 'Port', '7');
      |             set_param([gcb '/f32IntegPartK_1FW_Out'], 'Port', '8');
      |             set_param([gcb '/f32InK_1FW_Out'], 'Port', '9');
      |             set_param([gcb '/f32State_Out'], 'Port', '10');
      |         end
      | 
      |         set_param(gcb,'MaskEnables',{'on','on','on','off','off','off','off','off','off','off','off','off','off','off','off','off','off','off','off'});
      | 
      |         if (posblk(4) - posblk(2)) < 875
      |           height = 875;
      |           set_param(gcb,'Position',[posblk(1), posblk(2), posblk(3), posblk(2)+height])
      |         end
      |     else
      |         if (showDebugOutputs == 2) && (strcmp(get_param([gcb '/f32WReqFilt'], 'BlockType'), 'Terminator'))
      |             % shown debugging outputs
      |             pos = get_param(    [gcb '/f32WReqFilt'], 'Position');
      |             orient = get_param( [gcb '/f32WReqFilt'], 'Orientation');
      |             delete_block(       [gcb '/f32WReqFilt']);
      |             add_block('built-in/Outport', [gcb '/f32WReqFilt'], 'Position', pos, 'Orientation', orient);
      | 
      |             pos = get_param(    [gcb '/f32WErr'], 'Position');
      |             orient = get_param( [gcb '/f32WErr'], 'Orientation');
      |             delete_block(       [gcb '/f32WErr']);
      |             add_block('built-in/Outport', [gcb '/f32WErr'], 'Position', pos, 'Orientation', orient);
      | 
      |             pos = get_param(    [gcb '/f32WFbckFilt'], 'Position');
      |             orient = get_param( [gcb '/f32WFbckFilt'], 'Orientation');
      |             delete_block(       [gcb '/f32WFbckFilt']);
      |             add_block('built-in/Outport', [gcb '/f32WFbckFilt'], 'Position', pos, 'Orientation', orient);
      | 
      |             pos = get_param(    [gcb '/f32IDQReqAmp'], 'Position');
      |             orient = get_param( [gcb '/f32IDQReqAmp'], 'Orientation');
      |             delete_block(       [gcb '/f32IDQReqAmp']);
      |             add_block('built-in/Outport', [gcb '/f32IDQReqAmp'], 'Position', pos, 'Orientation', orient);
      | 
      |             pos = get_param(    [gcb '/f32IQErrSign'], 'Position');
      |             orient = get_param( [gcb '/f32IQErrSign'], 'Orientation');
      |             delete_block(       [gcb '/f32IQErrSign']);
      |             add_block('built-in/Outport', [gcb '/f32IQErrSign'], 'Position', pos, 'Orientation', orient);
      | 
      |             pos = get_param(    [gcb '/f32IQErr'], 'Position');
      |             orient = get_param( [gcb '/f32IQErr'], 'Orientation');
      |             delete_block(       [gcb '/f32IQErr']);
      |             add_block('built-in/Outport', [gcb '/f32IQErr'], 'Position', pos, 'Orientation', orient);
      | 
      |             pos = get_param(    [gcb '/f32FWErr'], 'Position');
      |             orient = get_param( [gcb '/f32FWErr'], 'Orientation');
      |             delete_block(       [gcb '/f32FWErr']);
      |             add_block('built-in/Outport', [gcb '/f32FWErr'], 'Position', pos, 'Orientation', orient);
      | 
      |             pos = get_param(    [gcb '/f32UQErr'], 'Position');
      |             orient = get_param( [gcb '/f32UQErr'], 'Orientation');
      |             delete_block(       [gcb '/f32UQErr']);
      |             add_block('built-in/Outport', [gcb '/f32UQErr'], 'Position', pos, 'Orientation', orient);
      | 
      |             pos = get_param(    [gcb '/f32FWErrFilt'], 'Position');
      |             orient = get_param( [gcb '/f32FWErrFilt'], 'Orientation');
      |             delete_block(       [gcb '/f32FWErrFilt']);
      |             add_block('built-in/Outport', [gcb '/f32FWErrFilt'], 'Position', pos, 'Orientation', orient);
      | 
      |             pos = get_param(    [gcb '/f32FWAngle'], 'Position');
      |             orient = get_param( [gcb '/f32FWAngle'], 'Orientation');
      |             delete_block(       [gcb '/f32FWAngle']);
      |             add_block('built-in/Outport', [gcb '/f32FWAngle'], 'Position', pos, 'Orientation', orient);
      | 
      |             pos = get_param(    [gcb '/f32FWSin'], 'Position');
      |             orient = get_param( [gcb '/f32FWSin'], 'Orientation');
      |             delete_block(       [gcb '/f32FWSin']);
      |             add_block('built-in/Outport', [gcb '/f32FWSin'], 'Position', pos, 'Orientation', orient);
      | 
      |             pos = get_param(    [gcb '/f32FWCos'], 'Position');
      |             orient = get_param( [gcb '/f32FWCos'], 'Orientation');
      |             delete_block(       [gcb '/f32FWCos']);
      |             add_block('built-in/Outport', [gcb '/f32FWCos'], 'Position', pos, 'Orientation', orient);
      | 
      |             set_param([gcb '/pIDQReq'], 'Port', '1');
      |             set_param([gcb '/u16LimitFlagQ'], 'Port', '2');
      |             set_param([gcb '/u16LimitFlagFW'], 'Port', '3');
      |             set_param([gcb '/f32WReqFilt'], 'Port', '4');
      |             set_param([gcb '/f32WErr'], 'Port', '5');
      |             set_param([gcb '/f32WFbckFilt'], 'Port', '6');
      |             set_param([gcb '/f32IDQReqAmp'], 'Port', '7');
      |             set_param([gcb '/f32IQErrSign'], 'Port', '8');
      |             set_param([gcb '/f32IQErr'], 'Port', '9');
      |             set_param([gcb '/f32FWErr'], 'Port', '10');
      |             set_param([gcb '/f32UQErr'], 'Port', '11');
      |             set_param([gcb '/f32FWErrFilt'], 'Port', '12');
      |             set_param([gcb '/f32FWAngle'], 'Port', '13');
      |             set_param([gcb '/f32FWSin'], 'Port', '14');
      |             set_param([gcb '/f32FWCos'], 'Port', '15');
      |             set_param([gcb '/f32AccW_Out'], 'Port', '16');
      |             set_param([gcb '/f32AccFW_Out'], 'Port', '17');
      |             set_param([gcb '/f32IntegPartK_1Q_Out'], 'Port', '18');
      |             set_param([gcb '/f32InK_1Q_Out'], 'Port', '19');
      |             set_param([gcb '/f32IntegPartK_1FW_Out'], 'Port', '20');
      |             set_param([gcb '/f32InK_1FW_Out'], 'Port', '21');
      |             set_param([gcb '/f32State_Out'], 'Port', '22');
      |         elseif (showDebugOutputs == 1) && (strcmp(get_param([gcb '/f32WReqFilt'], 'BlockType'), 'Outport'))
      |             % hidden debugging outputs
      |             pos = get_param(    [gcb '/f32WReqFilt'], 'Position');
      |             orient = get_param( [gcb '/f32WReqFilt'], 'Orientation');
      |             delete_block(       [gcb '/f32WReqFilt']);
      |             add_block('built-in/Terminator', [gcb '/f32WReqFilt'], 'Position', pos, 'Orientation', orient);
      | 
      |             pos = get_param(    [gcb '/f32WErr'], 'Position');
      |             orient = get_param( [gcb '/f32WErr'], 'Orientation');
      |             delete_block(       [gcb '/f32WErr']);
      |             add_block('built-in/Terminator', [gcb '/f32WErr'], 'Position', pos, 'Orientation', orient);
      | 
      |             pos = get_param(    [gcb '/f32WFbckFilt'], 'Position');
      |             orient = get_param( [gcb '/f32WFbckFilt'], 'Orientation');
      |             delete_block(       [gcb '/f32WFbckFilt']);
      |             add_block('built-in/Terminator', [gcb '/f32WFbckFilt'], 'Position', pos, 'Orientation', orient);
      | 
      |             pos = get_param(    [gcb '/f32IDQReqAmp'], 'Position');
      |             orient = get_param( [gcb '/f32IDQReqAmp'], 'Orientation');
      |             delete_block(       [gcb '/f32IDQReqAmp']);
      |             add_block('built-in/Terminator', [gcb '/f32IDQReqAmp'], 'Position', pos, 'Orientation', orient);
      | 
      |             pos = get_param(    [gcb '/f32IQErrSign'], 'Position');
      |             orient = get_param( [gcb '/f32IQErrSign'], 'Orientation');
      |             delete_block(       [gcb '/f32IQErrSign']);
      |             add_block('built-in/Terminator', [gcb '/f32IQErrSign'], 'Position', pos, 'Orientation', orient);
      | 
      |             pos = get_param(    [gcb '/f32IQErr'], 'Position');
      |             orient = get_param( [gcb '/f32IQErr'], 'Orientation');
      |             delete_block(       [gcb '/f32IQErr']);
      |             add_block('built-in/Terminator', [gcb '/f32IQErr'], 'Position', pos, 'Orientation', orient);
      | 
      |             pos = get_param(    [gcb '/f32FWErr'], 'Position');
      |             orient = get_param( [gcb '/f32FWErr'], 'Orientation');
      |             delete_block(       [gcb '/f32FWErr']);
      |             add_block('built-in/Terminator', [gcb '/f32FWErr'], 'Position', pos, 'Orientation', orient);
      | 
      |             pos = get_param(    [gcb '/f32UQErr'], 'Position');
      |             orient = get_param( [gcb '/f32UQErr'], 'Orientation');
      |             delete_block(       [gcb '/f32UQErr']);
      |             add_block('built-in/Terminator', [gcb '/f32UQErr'], 'Position', pos, 'Orientation', orient);
      | 
      |             pos = get_param(    [gcb '/f32FWErrFilt'], 'Position');
      |             orient = get_param( [gcb '/f32FWErrFilt'], 'Orientation');
      |             delete_block(       [gcb '/f32FWErrFilt']);
      |             add_block('built-in/Terminator', [gcb '/f32FWErrFilt'], 'Position', pos, 'Orientation', orient);
      | 
      |             pos = get_param(    [gcb '/f32FWAngle'], 'Position');
      |             orient = get_param( [gcb '/f32FWAngle'], 'Orientation');
      |             delete_block(       [gcb '/f32FWAngle']);
      |             add_block('built-in/Terminator', [gcb '/f32FWAngle'], 'Position', pos, 'Orientation', orient);
      | 
      |             pos = get_param(    [gcb '/f32FWSin'], 'Position');
      |             orient = get_param( [gcb '/f32FWSin'], 'Orientation');
      |             delete_block(       [gcb '/f32FWSin']);
      |             add_block('built-in/Terminator', [gcb '/f32FWSin'], 'Position', pos, 'Orientation', orient);
      | 
      |             pos = get_param(    [gcb '/f32FWCos'], 'Position');
      |             orient = get_param( [gcb '/f32FWCos'], 'Orientation');
      |             delete_block(       [gcb '/f32FWCos']);
      |             add_block('built-in/Terminator', [gcb '/f32FWCos'], 'Position', pos, 'Orientation', orient);
      | 
      |             set_param([gcb '/pIDQReq'], 'Port', '1');
      |             set_param([gcb '/u16LimitFlagQ'], 'Port', '2');
      |             set_param([gcb '/u16LimitFlagFW'], 'Port', '3');
      |             set_param([gcb '/f32AccW_Out'], 'Port', '4');
      |             set_param([gcb '/f32AccFW_Out'], 'Port', '5');
      |             set_param([gcb '/f32IntegPartK_1Q_Out'], 'Port', '6');
      |             set_param([gcb '/f32InK_1Q_Out'], 'Port', '7');
      |             set_param([gcb '/f32IntegPartK_1FW_Out'], 'Port', '8');
      |             set_param([gcb '/f32InK_1FW_Out'], 'Port', '9');
      |             set_param([gcb '/f32State_Out'], 'Port', '10');
      |         end
      |     end
      | end
      settings: RTWSystemCode=Inline
      mask TypeOptions showStates: Hide (faster execution) | Show (allows debugging; connect feedback loops manually)
      mask Callback showStates:
      | maskStr = get_param(gcb,'showStates');
      | if strcmp(maskStr,'Hide (faster execution)'),
      |     set_param(gcb,'MaskEnables',{'on','on','off','on','on','on','on','on','on','on','on','on','on','on','on','on','on','on','on'});
      | else
      |     set_param(gcb,'MaskEnables',{'on','on','on','off','off','off','off','off','off','off','off','off','off','off','off','off','off','off','off'});
      | end
      mask TypeOptions resetStatesEnable: Pre-set according to the first set of inputs after reset | Clear to zero
      mask TypeOptions showDebugOutputs: Hide | Show
      mask Display:
      | color('black');
      | pos = get_param(gcb, 'Position');
      | width = pos(3) - pos(1);
      | height = pos(4) - pos(2);
      | tX=width/2;
      | tY=height - 25;
      | color('black');
      | text(tX,tY, 'AMCLIB_FWSpeedLoop_F32', 'horizontalAlignment', 'center');
      | if showStates == 2
      |   color('red');
      |   text(tX,tY - 20, ['debugging mode' char(13) char(10) '(limited performance)'], 'horizontalAlignment', 'center');
      | end
